simulink model "S12_hellcat_2022_stock_v11"  (R2026a)
settings: Solver=FixedStepDiscrete  StopTime=90  FixedStep=0.02
undefined symbols (not defined in the file): s12_v11_model_excitation_afterfire_step, s12_v11_model_ptr_controls_step, s12_v11_model_renderer_gain_step, s12_v11_model_stereo_renderer_step, s12_v11_model_vehicle_state_step
settings Model: Creator=Jovi  LastModifiedBy=Jovi

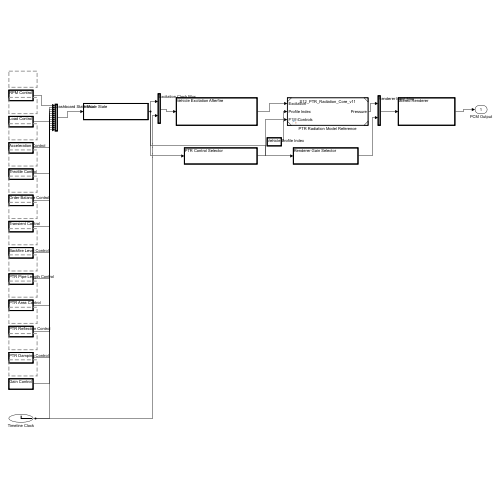
[thumbnail: Simulink's stored preview of the top-level diagram]
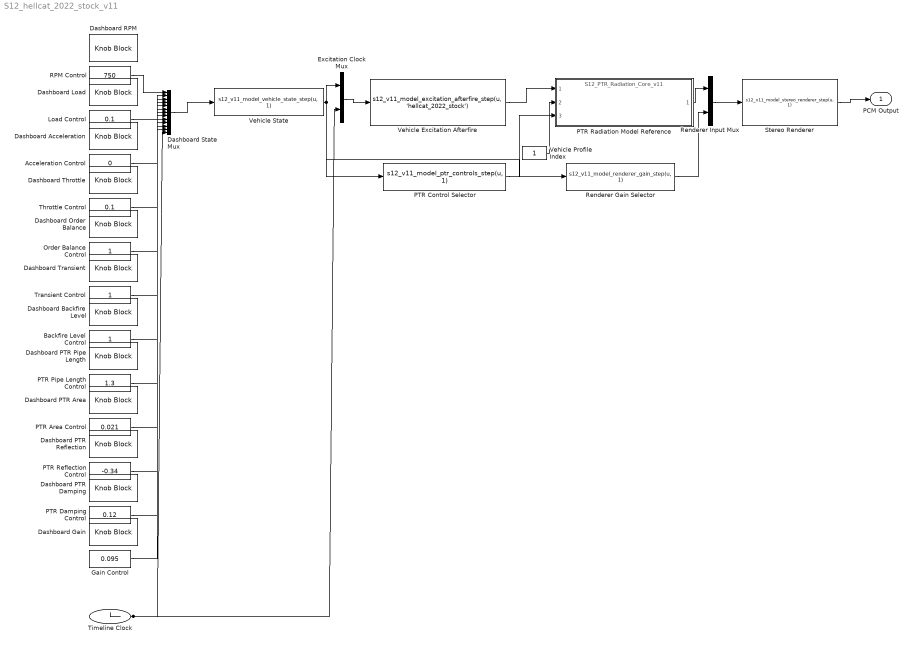
== system S12_hellcat_2022_stock_v11 ==
  Acceleration Control : Constant  Value=0  SampleTime=0.02
  Backfire Level Control : Constant  SampleTime=0.02
  Dashboard Acceleration : KnobBlock  ScaleMin=-4  ScaleMax=8  TickInterval=0.12
  Dashboard Backfire Level : KnobBlock  ScaleMax=2  TickInterval=0.02
  Dashboard Gain : KnobBlock  ScaleMax=0.20000000000000001  TickInterval=0.002
  Dashboard Load : KnobBlock  ScaleMax=1  TickInterval=0.01
  Dashboard Order Balance : KnobBlock  ScaleMax=2  TickInterval=0.02
  Dashboard PTR Area : KnobBlock  ScaleMin=0.0050000000000000001  ScaleMax=0.050000000000000003  TickInterval=0.00045000000000000004
  Dashboard PTR Damping : KnobBlock  ScaleMin=0.01  ScaleMax=0.5  TickInterval=0.0048999999999999998
  Dashboard PTR Pipe Length : KnobBlock  ScaleMin=0.5  ScaleMax=2  TickInterval=0.014999999999999999
  Dashboard PTR Reflection : KnobBlock  ScaleMin=-0.90000000000000002  ScaleMax=0.20000000000000001  TickInterval=0.011000000000000001
  Dashboard RPM : KnobBlock  ScaleMin=600  ScaleMax=10000  TickInterval=94
  Dashboard State Mux : Mux  Inputs=13
  Dashboard Throttle : KnobBlock  ScaleMax=1  TickInterval=0.01
  Dashboard Transient : KnobBlock  ScaleMax=2  TickInterval=0.02
  Excitation Clock Mux : Mux  Inputs=2
  Gain Control : Constant  Value=0.095  SampleTime=0.02
  Load Control : Constant  Value=0.1  SampleTime=0.02
  Order Balance Control : Constant  SampleTime=0.02
  PTR Area Control : Constant  Value=0.021  SampleTime=0.02
  PTR Control Selector : MATLABFcn  MATLABFcn=s12_v11_model_ptr_controls_step(u, 1)  OutputDimensions=[4 1]  Output1D=off
  PTR Damping Control : Constant  Value=0.12  SampleTime=0.02
  PTR Pipe Length Control : Constant  Value=1.3  SampleTime=0.02
  PTR Radiation Model Reference : ModelReference  ModelNameDialog=S12_PTR_Radiation_Core_v11  SimulationMode=Normal  ModelReferenceVersion=1.8
  PTR Reflection Control : Constant  Value=-0.34  SampleTime=0.02
  RPM Control : Constant  Value=750  SampleTime=0.02
  Renderer Gain Selector : MATLABFcn  MATLABFcn=s12_v11_model_renderer_gain_step(u, 1)  OutputDimensions=[1 1]  Output1D=off
  Renderer Input Mux : Mux  Inputs=2
  Stereo Renderer : MATLABFcn  MATLABFcn=s12_v11_model_stereo_renderer_step(u, 1)  OutputDimensions=[960 2]  Output1D=off
  Throttle Control : Constant  Value=0.1  SampleTime=0.02
  Timeline Clock : Clock
  Transient Control : Constant  SampleTime=0.02
  Vehicle Excitation Afterfire : MATLABFcn  MATLABFcn=s12_v11_model_excitation_afterfire_step(u, 'hellcat_2022_stock')  OutputDimensions=[960 1]  Output1D=off
  Vehicle Profile Index : Constant  SampleTime=0.02
  Vehicle State : MATLABFcn  MATLABFcn=s12_v11_model_vehicle_state_step(u, 1)  OutputDimensions=[21 1]  Output1D=off
  PCM Output : Outport
  wires:
  RPM Control/1 -> Dashboard State Mux/1
  Load Control/1 -> Dashboard State Mux/2
  Acceleration Control/1 -> Dashboard State Mux/3
  Throttle Control/1 -> Dashboard State Mux/4
  Order Balance Control/1 -> Dashboard State Mux/5
  Transient Control/1 -> Dashboard State Mux/6
  Backfire Level Control/1 -> Dashboard State Mux/7
  PTR Pipe Length Control/1 -> Dashboard State Mux/8
  PTR Area Control/1 -> Dashboard State Mux/9
  PTR Reflection Control/1 -> Dashboard State Mux/10
  PTR Damping Control/1 -> Dashboard State Mux/11
  Gain Control/1 -> Dashboard State Mux/12
  Timeline Clock/1 -> Dashboard State Mux/13, Excitation Clock Mux/2
  Dashboard State Mux/1 -> Vehicle State/1
  Vehicle State/1 -> Excitation Clock Mux/1, PTR Control Selector/1, Renderer Gain Selector/1
  Excitation Clock Mux/1 -> Vehicle Excitation Afterfire/1
  Vehicle Excitation Afterfire/1 -> PTR Radiation Model Reference/1
  Vehicle Profile Index/1 -> PTR Radiation Model Reference/2
  PTR Control Selector/1 -> PTR Radiation Model Reference/3
  PTR Radiation Model Reference/1 -> Renderer Input Mux/1
  Renderer Gain Selector/1 -> Renderer Input Mux/2
  Renderer Input Mux/1 -> Stereo Renderer/1
  Stereo Renderer/1 -> PCM Output/1
